simulink model "zhuangtaifankui1"  (R2022b)
settings: Solver=VariableStepAuto  StartTime=0.0  StopTime=10.0  RelTol=1e-3
settings Model: Creator=HONOR  LastModifiedBy=acer
settings DebuggingCC: UnconnectedInputMsg=warning  UnconnectedOutputMsg=warning  UnconnectedLineMsg=warning
settings ModelReferenceCC: EnableRefExpFcnMdlSchedulingChecks=on
settings RTWCC: DLArmComputeVersion=19.05

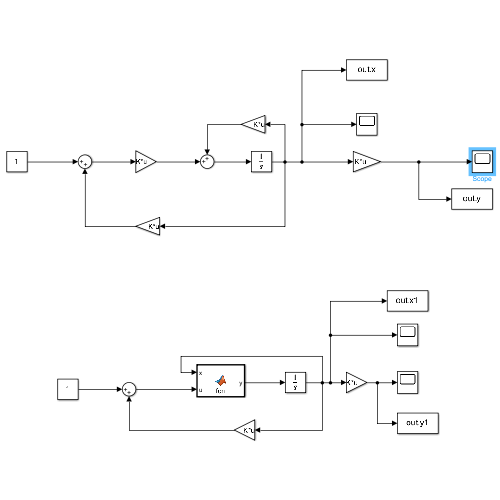
[thumbnail: Simulink's stored preview of the top-level diagram]
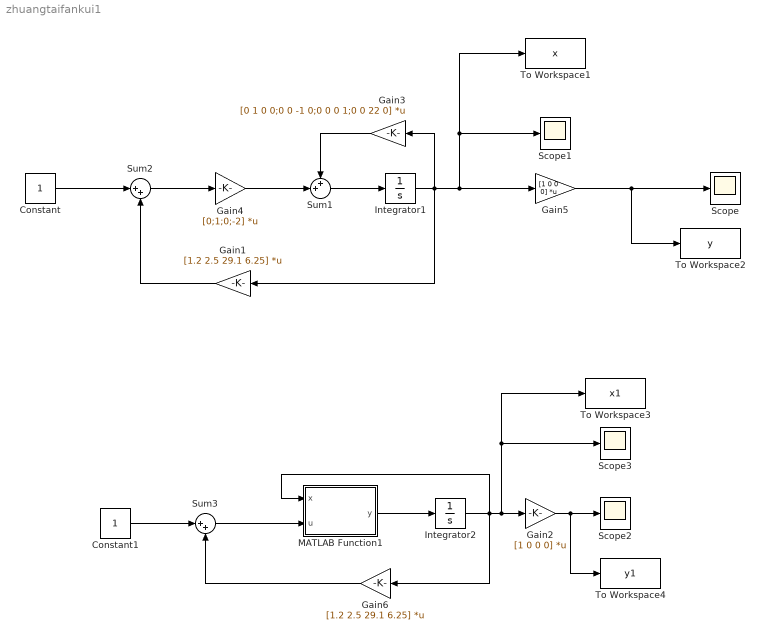
== system zhuangtaifankui1 ==
  Constant : Constant
  Constant1 : Constant
  Gain1 : Gain  Gain=[1.2 2.5 29.1 6.25]  Multiplication=Matrix(K*u)
  Gain2 : Gain  Gain=[1 0 0 0]  Multiplication=Matrix(K*u)
  Gain3 : Gain  Gain=[0 1 0 0;0 0 -1 0;0 0 0 1;0 0 22 0]  Multiplication=Matrix(K*u)
  Gain4 : Gain  Gain=[0;1;0;-2]  Multiplication=Matrix(K*u)
  Gain5 : Gain  Gain=[1 0 0 0]  Multiplication=Matrix(K*u)
  Gain6 : Gain  Gain=[1.2 2.5 29.1 6.25]  Multiplication=Matrix(K*u)
  Integrator1 : Integrator  InitialCondition=[0,0,0.1,0]
  Integrator2 : Integrator  InitialCondition=[0,0,0.1,0]
  MATLAB Function1 : MATLAB Function  TreatAsAtomicUnit=on
  Scope{,1..3} (4 alike) : Scope
  Sum1 : Sum  Inputs=++|
  Sum2 : Sum  Inputs=|++
  Sum3 : Sum  Inputs=|++
  To Workspace1 : ToWorkspace  VariableName=x  SaveFormat=Structure With Time  SampleTime=-1
  To Workspace2 : ToWorkspace  VariableName=y  SaveFormat=Structure With Time  SampleTime=-1
  To Workspace3 : ToWorkspace  VariableName=x1  SaveFormat=Structure With Time  SampleTime=-1
  To Workspace4 : ToWorkspace  VariableName=y1  SaveFormat=Structure With Time  SampleTime=-1
  wires:
  Gain5/1 -> Scope/1, To Workspace2/1
  Gain4/1 -> Sum1/2
  Sum1/1 -> Integrator1/1
  Integrator1/1 -> Gain5/1, To Workspace1/1, Scope1/1, Gain3/1, Gain1/1
  Gain3/1 -> Sum1/1
  Gain1/1 -> Sum2/2
  Constant/1 -> Sum2/1
  Sum2/1 -> Gain4/1
  MATLAB Function1/1(y) -> Integrator2/1
  Integrator2/1 -> Gain6/1, MATLAB Function1/1(x), To Workspace3/1, Scope3/1, Gain2/1
  Gain2/1 -> To Workspace4/1, Scope2/1
  Sum3/1 -> MATLAB Function1/2(u)
  Constant1/1 -> Sum3/1
  Gain6/1 -> Sum3/2

== matlab function zhuangtaifankui1/MATLAB Function1 ==
  data: x input; u input; y output
function y = fcn(x, u)
M=1;
m=0.1;
l=0.5;
g=10;
Dx3=x(4);
Dx4=(u*cos(x(3))-(M+m)*g*sin(x(3))+m*l*sin(x(3))*cos(x(3)*x(4)))/(m*l*cos(x(3))*cos(x(3))-(M+m)*l);
Dx1=x(2);
Dx2=((u+m*l*sin(x(3)*x(4)*x(4))-m*g*cos(x(3))*sin(x(3)))/(M+m-m*cos(x(3))*cos(x(3))));
y=[Dx1;Dx2;Dx3;Dx4];
